simulink model "pendulum"  (R2024b)
settings: Solver=VariableStepAuto  StartTime=0.0  StopTime=3  RelTol=1e-3
values from neighbouring files (symbols this model uses):
  K = lqr(A,B,Q,R)    [Rotary_Pendulum_Parameters.m]
  r = [0; pi; 0; 0]    [Rotary_Pendulum_Parameters.m]
  x0 = [0; 0.1; 0; 0]    [Rotary_Pendulum_Parameters.m]
libraries: simulink_extras x4
settings Model: Creator=geehoonjung  LastModifiedBy=geehoonjung

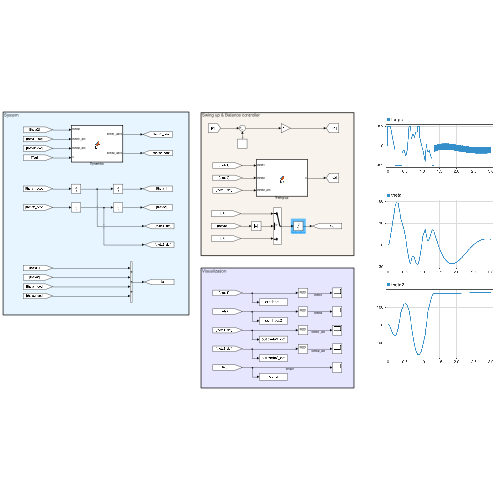
[thumbnail: Simulink's stored preview of the top-level diagram]
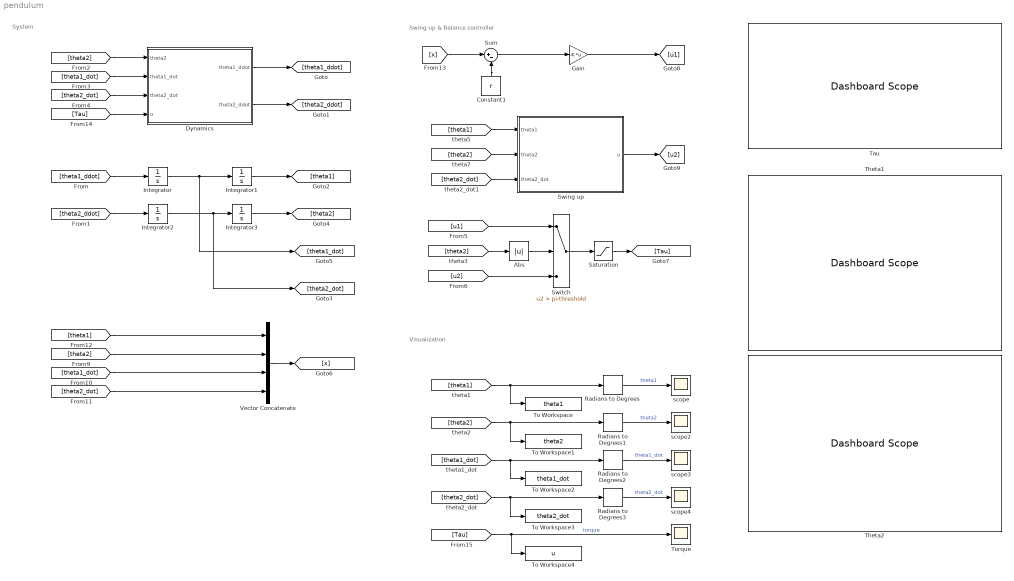
== system pendulum ==
  note: Swing up & Balance controller
  note: System
  note: Visualization
  Abs : Abs  SaturateOnIntegerOverflow=off
  Constant1 : Constant  Value=r
  Dynamics : MATLAB Function  TreatAsAtomicUnit=on
  Gain : Gain  Gain=-K  Multiplication=Matrix(K*u)
  Integrator : Integrator  InitialCondition=x0(3)
  Integrator1 : Integrator  InitialCondition=x0(1)
  Integrator2 : Integrator  InitialCondition=x0(4)
  Integrator3 : Integrator  InitialCondition=x0(2)
  Radians to Degrees{,1..3} (4 alike) : simulink_extras/Transformations/Radians to Degrees
  Saturation : Saturate  UpperLimit=0.2  LowerLimit=-0.2
  Sum : Sum  Inputs=|+-
  Swing up : MATLAB Function  TreatAsAtomicUnit=on
  Switch : Switch  Criteria=u2 > Threshold  Threshold=pi-threshold  SaturateOnIntegerOverflow=off  InputSameDT=off
  Tau : DashboardScope
  Theta1 : DashboardScope
  Theta2 : DashboardScope
  To Workspace : ToWorkspace  VariableName=theta1  SaveFormat=Timeseries  SampleTime=-1
  To Workspace1 : ToWorkspace  VariableName=theta2  SaveFormat=Timeseries  SampleTime=-1
  To Workspace2 : ToWorkspace  VariableName=theta1_dot  SaveFormat=Timeseries  SampleTime=-1
  To Workspace3 : ToWorkspace  VariableName=theta2_dot  SaveFormat=Timeseries  SampleTime=-1
  To Workspace4 : ToWorkspace  VariableName=u  SaveFormat=Timeseries  SampleTime=-1
  Torque : Scope
  Vector Concatenate : Concatenate  NumInputs=4
  scope{,2..4} (4 alike) : Scope
  wires:
  Dynamics/1(theta1_ddot) -> [theta1_ddot]
  Dynamics/2(theta2_ddot) -> [theta2_ddot]
  [theta1_ddot] -> Integrator/1
  Integrator/1 -> Integrator1/1, [theta1_dot]
  [theta2_ddot] -> Integrator2/1
  Integrator2/1 -> Integrator3/1, [theta2_dot]
  [theta2] -> Dynamics/1(theta2)
  [theta1_dot] -> Dynamics/2(theta1_dot)
  [theta2_dot] -> Dynamics/3(theta2_dot)
  Integrator3/1 -> [theta2]
  Integrator1/1 -> [theta1]
  [theta2] -> Radians to Degrees1/1, To Workspace1/1
  [theta1_dot] -> Radians to Degrees2/1, To Workspace2/1
  [theta2_dot] -> Radians to Degrees3/1, To Workspace3/1
  [theta2] -> Vector Concatenate/2
  [theta1] -> Vector Concatenate/1
  [theta1_dot] -> Vector Concatenate/3
  [theta2_dot] -> Vector Concatenate/4
  Vector Concatenate/1 -> [x]
  Constant1/1 -> Sum/2
  Sum/1 -> Gain/1
  [Tau] -> Dynamics/4(u)
  [Tau] -> To Workspace4/1, Torque/1  "torque"
  [theta2] -> Swing up/2(theta2)
  [theta2_dot] -> Swing up/3(theta2_dot)
  Saturation/1 -> [Tau]
  Switch/1 -> Saturation/1
  [theta2] -> Abs/1
  [theta1] -> Swing up/1(theta1)
  Gain/1 -> [u1]
  Swing up/1(u) -> [u2]
  [x] -> Sum/1
  Abs/1 -> Switch/2
  [u1] -> Switch/1
  [u2] -> Switch/3
  [theta1] -> Radians to Degrees/1, To Workspace/1
  Radians to Degrees/1 -> scope/1  "theta1"
  Radians to Degrees1/1 -> scope2/1  "theta2"
  Radians to Degrees2/1 -> scope3/1  "theta1_dot"
  Radians to Degrees3/1 -> scope4/1  "theta2_dot"

== matlab function pendulum/Swing up ==
  data: theta1 input; theta2 input; u output; theta2_dot input
function u = fcn(theta1, theta2, theta2_dot)

theta2 = theta2 - pi;

g = 9.81;
L2 = 0.08;
l2 = 0.5*L2;
m2 = 0.128;
I2 = m2*L2^2/12;
J2 = I2 + m2*l2^2;

KE = 3;
E0 = 2*m2*g*l2;

E = 0.5*J2*(theta2_dot^2) + m2*g*l2*(1+cos(theta2));
s = sign(theta2_dot*cos(theta2));
u = KE*(E0 - E)*s - 0.3 * theta1;

== matlab function pendulum/Dynamics ==
  data: theta2 input; theta1_dot input; theta2_dot input; u input; theta1_ddot output; theta2_ddot output
function [theta1_ddot, theta2_ddot] = fcn(theta2, theta1_dot, theta2_dot, u)

g = 9.81;

m1 = 0.257; % Mass of rotary arm with two thum screws
m2 = 0.127; % Mass of pendulum

L1 = 0.15; % Rotary arm length from pivot to tip
l1 = 0.5*L1; % Rotary arm length from pivot to center of mass 

L2 = 0.129; % Total length of pendulum
l2 = 0.5*L2; % Distance between center of mass and pivot of pendulum

J0 = 0;
I1 = m1*L1^2/12; % Rotary arm moment of inertia about its center of mass 
I2 = m2*L2^2/12; % Pendulum moment of inertia about center of mass 
J1 = I1 + m1*l1^2; % Rotary arm moment of inertia about pivot
J2 = I2 + m2*l2^2; % Pendulum moment of inertia about pivot

% Friction coefficients are approximated
d1 = 1e-3;
d2 = 1e-5;

M = [J0+J1+m2*L1^2+J2*sin(theta2)^2 m2*L1*l2*cos(theta2);
     m2*L1*l2*cos(theta2) J2];
V = [-m2*L1*l2*theta2_dot^2*sin(theta2) + J2*theta1_dot*theta2_dot*sin(2*theta2);
     -J2*theta1_dot^2*sin(theta2)*cos(theta2)];
G = [0; m2*g*l2*sin(theta2)];
D = [d1 0; d2 0];
B = [1; 0];
Tau = [u 0];

theta_ddot = M \ (-V - D * [theta1_dot; theta2_dot] - G + B * Tau);

theta1_ddot = theta_ddot(1);
theta2_ddot = theta_ddot(2);
